simulink model "dc_ac"  (R2018a)
settings: Solver=FixedStepAuto  StartTime=0.0  StopTime=10.0  RelTol=1e-3
libraries: powerlib x7
settings Model: Creator=mstruong  LastModifiedBy=mstruong
settings SolverCC: AutoInsertRateTranBlk=on

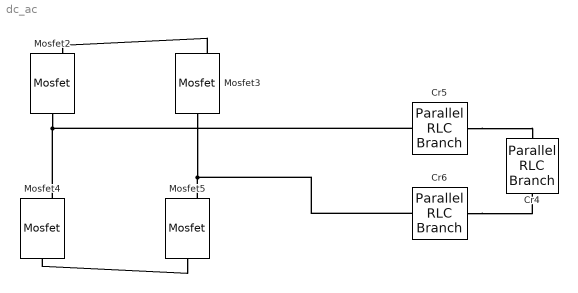
== system dc_ac ==
  Cr4 : powerlib/Elements/Parallel RLC Branch  LConnTagsString=a  RConnTagsString=__new0  BranchType=R  Resistance=1e6  Inductance=2.6e-6  SetiL0=off  InitialCurrent=0  Capacitance=2.4e-6  Setx0=off  InitialVoltage=0  Measurements=None
  Cr5 : powerlib/Elements/Parallel RLC Branch  LConnTagsString=a  RConnTagsString=__new0  BranchType=L  Resistance=1  Inductance=15e-6  SetiL0=off  InitialCurrent=0  Capacitance=2.4e-6  Setx0=off  InitialVoltage=0  Measurements=None
  Cr6 : powerlib/Elements/Parallel RLC Branch  LConnTagsString=a  RConnTagsString=__new0  BranchType=L  Resistance=1  Inductance=15e-6  SetiL0=off  InitialCurrent=0  Capacitance=2.4e-6  Setx0=off  InitialVoltage=0  Measurements=None
  Mosfet{2..5} (4 alike) : powerlib/Power Electronics/Mosfet  Ron=1.4  Lon=0  Rd=0.0000001  Vfd=1.5  IC=0  Rs=1e6  Cs=inf  Measurements=off
  wires:
  ? -> Mosfet3/1
  ? -> Mosfet5/1
  ? -> Mosfet2/1
  ? -> Mosfet4/1
  connections:
  Mosfet2/RConn1 -- Mosfet4/LConn1 -- Cr5/LConn1
  Cr6/LConn1 -- Mosfet5/LConn1 -- Mosfet3/RConn1
  Cr5/RConn1 -- Cr4/LConn1
  Cr6/RConn1 -- Cr4/RConn1
  Mosfet3/LConn1 -- Mosfet2/LConn1
  Mosfet5/RConn1 -- Mosfet4/RConn1
